simulink model "LMI_lema_6_statefeedback"  (Simulink 7.7)
settings: Solver=ode45  StartTime=0.0  StopTime=1900  RelTol=1e-3
values from neighbouring files (symbols this model uses):
  QT =     [FaseMinima.mat]    (also in FaseNaoMinima.mat; FaseNaoMinimaMudandoApenasGama.mat; settup.m = dynamics())
settings Model: Creator=Arthur  LastModifiedBy=Arthur

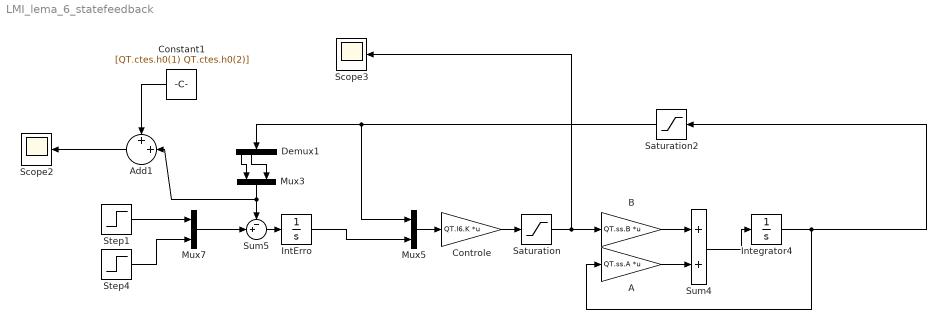
== system LMI_lema_6_statefeedback ==
  A : Gain  Gain=QT.ss.A  Multiplication=Matrix(K*u)
  Add1 : Sum  Inputs=++|
  B : Gain  Gain=QT.ss.B  Multiplication=Matrix(K*u)
  Constant1 : Constant  Value=[QT.ctes.h0(1) QT.ctes.h0(2)]
  Controle : Gain  Gain=QT.l6.K  Multiplication=Matrix(K*u)
  Demux1 : Demux
  IntErro : Integrator
  Integrator4 : Integrator
  Mux3 : Mux  Inputs=2
  Mux5 : Mux  Inputs=2
  Mux7 : Mux  Inputs=2
  Saturation : Saturate  UpperLimit=+1.5  LowerLimit=-1.5
  Saturation2 : Saturate  UpperLimit=10  LowerLimit=-5
  Scope2 : Scope
      settings: TimeRange=10  SaveName=Simulado
  Scope3 : Scope
      settings: TimeRange=3.947368421052632  YMin=1.005827505827506  YMax=3.346153846153847  SaveName=ScopeData2  SampleTime=0.3
  Step1 : Step  Time=300  SampleTime=0
  Step4 : Step  Time=1100  SampleTime=0
  Sum4 : Sum
  Sum5 : Sum  Inputs=-+|
  wires:
  A/1 -> Sum4/2
  B/1 -> Sum4/1
  Integrator4/1 -> A/1, Saturation2/1
  Sum4/1 -> Integrator4/1
  Controle/1 -> Saturation/1
  Mux5/1 -> Controle/1
  Sum5/1 -> IntErro/1
  Demux1/1 -> Mux3/1
  Demux1/2 -> Mux3/2
  Mux3/1 -> Sum5/1, Add1/2
  IntErro/1 -> Mux5/2
  Saturation/1 -> B/1, Scope3/1
  Saturation2/1 -> Demux1/1, Mux5/1
  Step1/1 -> Mux7/1
  Step4/1 -> Mux7/2
  Mux7/1 -> Sum5/2
  Add1/1 -> Scope2/1
  Constant1/1 -> Add1/1
